simulink model "PC_Quadcopter_Simulation_Hexacopter_health_wind"  (R2022b)
settings: Solver=ode4  StartTime=0.0  StopTime=100  FixedStep=0.01  MaxStep=0.06  RelTol=1e-3
PreLoadFcn:
  | DoB_parameter
model workspace (MAT data in the model file):
  Sig : Simulink.Signal (value not decoded)
values from neighbouring files (symbols this model uses):
  A = [ ... (first row only)    [DoB_parameter.m]
  B = [0 1 0]'    [DoB_parameter.m]
  C = [1 0 0]    [DoB_parameter.m]
  den_Inv_X = conv(num_X,den_Qfilter)    [DoB_parameter.m]
  den_Inv_Y = conv(num_Y, den_Qfilter)    [DoB_parameter.m]
  den_Inv_Z = conv(num_Z, den_Qfilter_Z)    [DoB_parameter.m]
  den_Qfilter = [1 a1/tau a0/tau^2]    [DoB_parameter.m]
  den_Qfilter_Z = [1 a1/tau a0/tau^2]    [DoB_parameter.m]
  I_xx = J(1,1)    [DoB_parameter.m]
  I_yy = J(2,2)    [DoB_parameter.m]
  I_zz = J(3,3)    [DoB_parameter.m]
  IC = block.DialogPrm(2).Data    [quadcopterDynamicsSFunction.m]
  L = [l1 l2 l3]'    [DoB_parameter.m]
  num_Inv_X = conv(den_X,num_Qfilter)    [DoB_parameter.m]
  num_Inv_Y = conv(den_Y, num_Qfilter)    [DoB_parameter.m]
  num_Inv_Z = conv(den_Z, num_Qfilter_Z)    [DoB_parameter.m]
  num_Qfilter = a0/tau^2    (= 100)    [DoB_parameter.m]
  num_Qfilter_Z = a0/tau^2    (= 11.1111111111)    [DoB_parameter.m]
undefined symbols (not defined in the file or in its folder): F, Light, magnitude, MIL, quadModel
libraries: simulink x37, sharedTrackingLibrary x1, aerolibwind2 x1
(part 3 of 3)

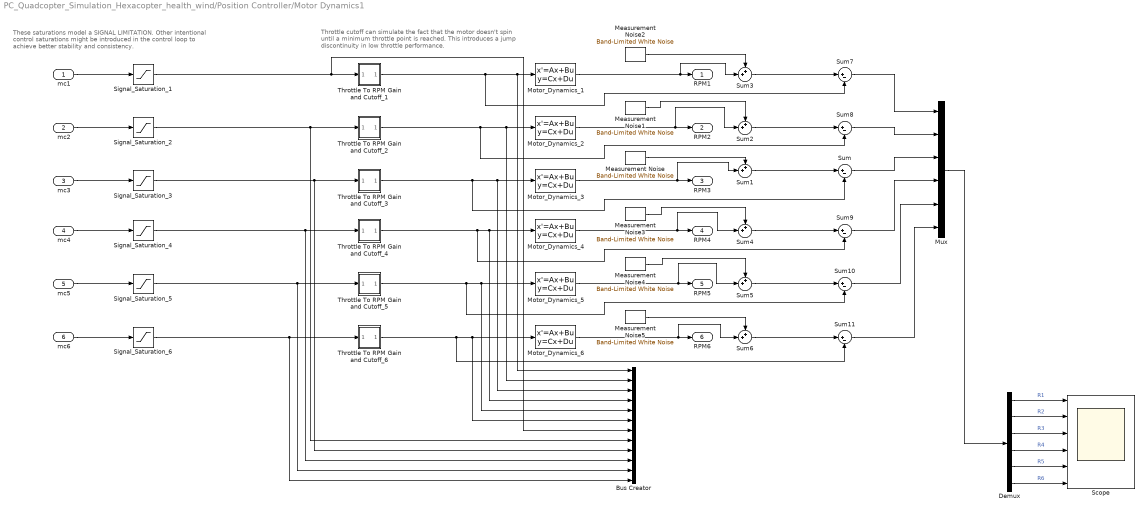
== system PC_Quadcopter_Simulation_Hexacopter_health_wind/Position Controller/Motor Dynamics1 ==
  note: These saturations model a SIGNAL LIMITATION.
      | Other intentional control saturations might be introduced in the
      | control loop to achieve better stability and consistency.
  note: Throttle cutoff can simulate the fact that the motor doesn't
      | spin until a minimum throttle point is reached. This introduces
      | a jump discontinuity in low throttle performance.
  mc1 : Inport
  mc2 : Inport  Port=2
  mc3 : Inport  Port=3
  mc4 : Inport  Port=4
  mc5 : Inport  Port=5
  mc6 : Inport  Port=6
  Bus Creator : BusCreator  Inputs=12
  Demux : Demux  Outputs=6
  Measurement Noise{,1..5} (6 alike) : simulink/Sources/Band-Limited White Noise  Cov=10^2  Ts=0.02  seed=[23342]
  Motor_Dynamics_1 : StateSpace  A=-1/quadModel.T  C=1/quadModel.T  D=0  InitialCondition=IC.w1*quadModel.T
  Motor_Dynamics_2 : StateSpace  A=-1/quadModel.T  C=1/quadModel.T  D=0  InitialCondition=IC.w2*quadModel.T
  Motor_Dynamics_3 : StateSpace  A=-1/quadModel.T  C=1/quadModel.T  D=0  InitialCondition=IC.w3*quadModel.T
  Motor_Dynamics_4 : StateSpace  A=-1/quadModel.T  C=1/quadModel.T  D=0  InitialCondition=IC.w4*quadModel.T
  Motor_Dynamics_5 : StateSpace  A=-1/quadModel.T  C=1/quadModel.T  D=0  InitialCondition=IC.w4*quadModel.T
  Motor_Dynamics_6 : StateSpace  A=-1/quadModel.T  C=1/quadModel.T  D=0  InitialCondition=IC.w4*quadModel.T
  Mux : Mux  Inputs=6
  Scope : Scope  NumInputPorts=6
  Signal_Saturation_{1..6} (6 alike) : Saturate  UpperLimit=100  LowerLimit=0
  Sum{,7..11} (6 alike) : Sum  Inputs=|+-
  Sum{1..6} (6 alike) : Sum  Inputs=++|
  Throttle To RPM Gain and Cutoff_1 : Subsystem
  Throttle To RPM Gain and Cutoff_2 : Subsystem
  Throttle To RPM Gain and Cutoff_3 : Subsystem
  Throttle To RPM Gain and Cutoff_4 : Subsystem
  Throttle To RPM Gain and Cutoff_5 : Subsystem
  Throttle To RPM Gain and Cutoff_6 : Subsystem
  RPM1 : Outport
  RPM2 : Outport  Port=2
  RPM3 : Outport  Port=3
  RPM4 : Outport  Port=4
  RPM5 : Outport  Port=5
  RPM6 : Outport  Port=6
  wires:
  Demux/1 -> Scope/1  "R1"
  Demux/2 -> Scope/2  "R2"
  Demux/3 -> Scope/3  "R3"
  Demux/4 -> Scope/4  "R4"
  Demux/5 -> Scope/5  "R5"
  Demux/6 -> Scope/6  "R6"
  Sum11/1 -> Mux/6
  Sum10/1 -> Mux/5
  Sum9/1 -> Mux/4
  Sum/1 -> Mux/3
  Sum8/1 -> Mux/2
  Sum7/1 -> Mux/1
  Sum6/1 -> Sum11/1
  Sum5/1 -> Sum10/1
  Sum4/1 -> Sum9/1
  Sum3/1 -> Sum7/1
  Sum2/1 -> Sum8/1
  Measurement Noise2/1 -> Sum3/1
  Measurement Noise1/1 -> Sum2/1
  Measurement Noise3/1 -> Sum4/1
  Measurement Noise4/1 -> Sum5/1
  Measurement Noise5/1 -> Sum6/1
  Sum1/1 -> Sum/1
  Measurement Noise/1 -> Sum1/1
  Mux/1 -> Demux/1
  Throttle To RPM Gain and Cutoff_6/1(Out5) -> Bus Creator/6, Motor_Dynamics_6/1, Sum11/2
  Signal_Saturation_6/1 -> Throttle To RPM Gain and Cutoff_6/1(In5), Bus Creator/12
  mc6/1 -> Signal_Saturation_6/1
  Motor_Dynamics_6/1 -> RPM6/1, Sum6/2
  Throttle To RPM Gain and Cutoff_5/1(Out5) -> Bus Creator/5, Motor_Dynamics_5/1, Sum10/2
  Signal_Saturation_5/1 -> Throttle To RPM Gain and Cutoff_5/1(In5), Bus Creator/11
  mc5/1 -> Signal_Saturation_5/1
  Motor_Dynamics_5/1 -> RPM5/1, Sum5/2
  Motor_Dynamics_4/1 -> RPM4/1, Sum4/2
  Motor_Dynamics_3/1 -> RPM3/1, Sum1/2
  Motor_Dynamics_2/1 -> RPM2/1, Sum2/2
  Motor_Dynamics_1/1 -> RPM1/1, Sum3/2
  Throttle To RPM Gain and Cutoff_4/1(Out5) -> Bus Creator/4, Motor_Dynamics_4/1, Sum9/2
  Throttle To RPM Gain and Cutoff_3/1(Out5) -> Bus Creator/3, Motor_Dynamics_3/1, Sum/2
  Throttle To RPM Gain and Cutoff_2/1(Out5) -> Bus Creator/2, Motor_Dynamics_2/1, Sum8/2
  Throttle To RPM Gain and Cutoff_1/1(Out5) -> Motor_Dynamics_1/1, Bus Creator/1, Sum7/2
  Signal_Saturation_4/1 -> Throttle To RPM Gain and Cutoff_4/1(In5), Bus Creator/10
  Signal_Saturation_3/1 -> Throttle To RPM Gain and Cutoff_3/1(In5), Bus Creator/9
  Signal_Saturation_2/1 -> Bus Creator/8, Throttle To RPM Gain and Cutoff_2/1(In5)
  Signal_Saturation_1/1 -> Throttle To RPM Gain and Cutoff_1/1(In5), Bus Creator/7
  mc3/1 -> Signal_Saturation_3/1
  mc2/1 -> Signal_Saturation_2/1
  mc4/1 -> Signal_Saturation_4/1
  mc1/1 -> Signal_Saturation_1/1

== system PC_Quadcopter_Simulation_Hexacopter_health_wind/Position Controller/Phi Command Control ==
  note: -1 Gain is required because a "negative"
      | angle of Phi induces a positive velocity
      | in the body frame y direction!
  Desired Yb Velocity : Inport
  Yb Velocity : Inport  Port=2
  Attitude Limits_Phi : Saturate  UpperLimit=ASat  LowerLimit=-ASat
  Gain : Gain  Gain=-1
  Kdp : Gain  Gain=Kd
  Kpp : Gain  Gain=Kp
  Sum3 : Sum  Inputs=|+-
  Sum6 : Sum  Inputs=|+-
  V Derivative : Derivative
  Phi_cmd : Outport
  wires:
  V Derivative/1 -> Kdp/1
  Attitude Limits_Phi/1 -> Phi_cmd/1  "Phi_cmd"
  Sum6/1 -> Gain/1
  Kpp/1 -> Sum6/1
  Sum3/1 -> Kpp/1  "Velocity Error"
  Yb Velocity/1 -> V Derivative/1, Sum3/2
  Desired Yb Velocity/1 -> Sum3/1
  Gain/1 -> Attitude Limits_Phi/1
  Kdp/1 -> Sum6/2

== system PC_Quadcopter_Simulation_Hexacopter_health_wind/Position Controller/Phi Command Control1 ==
  note: -1 Gain is required because a "negative"
      | angle of Phi induces a positive velocity
      | in the body frame y direction!
  Desired Yb Velocity : Inport
  Attitude Limits_Phi : Saturate  UpperLimit=ASat  LowerLimit=-ASat
  Gain : Gain  Gain=-1
  Kpp : Gain  Gain=Kp
  Phi_cmd : Outport
  wires:
  Gain/1 -> Attitude Limits_Phi/1
  Desired Yb Velocity/1 -> Kpp/1  "Velocity Error"
  Kpp/1 -> Gain/1
  Attitude Limits_Phi/1 -> Phi_cmd/1  "Phi_cmd"

== system PC_Quadcopter_Simulation_Hexacopter_health_wind/Position Controller/Phi Command Control2 ==
  note: -1 Gain is required because a "negative"
      | angle of Phi induces a positive velocity
      | in the body frame y direction!
  Desired Yb Velocity : Inport
  Yb Velocity : Inport  Port=2
  Attitude Limits_Phi : Saturate  UpperLimit=ASat  LowerLimit=-ASat
  Gain : Gain  Gain=-1
  Kdp : Gain  Gain=Kd
  Kpp : Gain  Gain=Kp
  Sum3 : Sum  Inputs=|+-
  Sum6 : Sum  Inputs=|+-
  V Derivative : Derivative
  Phi_cmd : Outport
  wires:
  Kdp/1 -> Sum6/2
  Gain/1 -> Attitude Limits_Phi/1
  Desired Yb Velocity/1 -> Sum3/1
  Yb Velocity/1 -> Sum3/2, V Derivative/1
  Sum3/1 -> Kpp/1  "Velocity Error"
  Kpp/1 -> Sum6/1
  Sum6/1 -> Gain/1
  Attitude Limits_Phi/1 -> Phi_cmd/1  "Phi_cmd"
  V Derivative/1 -> Kdp/1

== system PC_Quadcopter_Simulation_Hexacopter_health_wind/Position Controller/Pitch (Theta) Control ==
  Attitude Command : Inport
  Bus Selector : BusSelector  OutputSignals=The_cmd
  Integrator Limited : Integrator  LimitOutput=on  UpperSaturationLimit=USat  LowerSaturationLimit=LSat
  Kit : Gain  Gain=Kit
  Kpt : Gain  Gain=Kpt
  Sum1 : Sum  Inputs=++|
  Theta Correction : Outport
  wires:
  Attitude Command/1 -> Bus Selector/1
  Sum1/1 -> Theta Correction/1
  Kpt/1 -> Sum1/1  "P Corr"
  Kit/1 -> Sum1/2  "I Corr"
  Integrator Limited/1 -> Kit/1
  Bus Selector/1 -> Integrator Limited/1, Kpt/1  "<The_cmd>"

== system PC_Quadcopter_Simulation_Hexacopter_health_wind/Position Controller/Pitch (Theta) Control1 ==
  Attitude Command : Inport
  Bus Selector : BusSelector  OutputSignals=The_cmd
  Integrator Limited : Integrator  LimitOutput=on  UpperSaturationLimit=USat  LowerSaturationLimit=LSat
  Kit : Gain  Gain=Kit
  Kpt : Gain  Gain=Kpt
  Sum1 : Sum  Inputs=++|
  Theta Correction : Outport
  wires:
  Bus Selector/1 -> Kpt/1, Integrator Limited/1  "<The_cmd>"
  Integrator Limited/1 -> Kit/1
  Kit/1 -> Sum1/2  "I Corr"
  Kpt/1 -> Sum1/1  "P Corr"
  Sum1/1 -> Theta Correction/1
  Attitude Command/1 -> Bus Selector/1

== system PC_Quadcopter_Simulation_Hexacopter_health_wind/Position Controller/Roll (Phi) Control  ==
  "Attitude Command " : Inport
  Bus Selector : BusSelector  OutputSignals=Phi_cmd
  Integrator Limited : Integrator  LimitOutput=on  UpperSaturationLimit=USat  LowerSaturationLimit=LSat
  Kip : Gain  Gain=Kip
  Kpp : Gain  Gain=Kpp
  Sum1 : Sum  Inputs=++|
  Phi Correction : Outport
  wires:
  Sum1/1 -> Phi Correction/1
  Kpp/1 -> Sum1/1  "P Corr"
  Kip/1 -> Sum1/2  "I Corr"
  Integrator Limited/1 -> Kip/1
  "Attitude Command "/1 -> Bus Selector/1
  Bus Selector/1 -> Integrator Limited/1, Kpp/1  "<Phi_cmd>"

== system PC_Quadcopter_Simulation_Hexacopter_health_wind/Position Controller/Roll (Phi) Control 1 ==
  "Attitude Command " : Inport
  Bus Selector : BusSelector  OutputSignals=Phi_cmd
  Integrator Limited : Integrator  LimitOutput=on  UpperSaturationLimit=USat  LowerSaturationLimit=LSat
  Kip : Gain  Gain=Kip
  Kpp : Gain  Gain=Kpp
  Sum1 : Sum  Inputs=++|
  Phi Correction : Outport
  wires:
  Bus Selector/1 -> Kpp/1, Integrator Limited/1  "<Phi_cmd>"
  "Attitude Command "/1 -> Bus Selector/1
  Integrator Limited/1 -> Kip/1
  Kip/1 -> Sum1/2  "I Corr"
  Kpp/1 -> Sum1/1  "P Corr"
  Sum1/1 -> Phi Correction/1

== system PC_Quadcopter_Simulation_Hexacopter_health_wind/Position Controller/Theta Command Control ==
  Desired Xb Velocity : Inport
  Xb Velocity : Inport  Port=2
  Attitude Limits_Theta : Saturate  UpperLimit=ASat  LowerLimit=-ASat
  Kdt : Gain  Gain=Kd
  Kpt : Gain  Gain=Kp
  Sum3 : Sum  Inputs=|+-
  Sum6 : Sum  Inputs=|+-
  U Derivative : Derivative
  The_cmd : Outport
  wires:
  Kdt/1 -> Sum6/2
  U Derivative/1 -> Kdt/1
  Attitude Limits_Theta/1 -> The_cmd/1  "The_cmd"
  Sum6/1 -> Attitude Limits_Theta/1
  Kpt/1 -> Sum6/1
  Sum3/1 -> Kpt/1  "Velocity Error"
  Xb Velocity/1 -> U Derivative/1, Sum3/2
  Desired Xb Velocity/1 -> Sum3/1

== system PC_Quadcopter_Simulation_Hexacopter_health_wind/Position Controller/Theta Command Control1 ==
  Desired Xb Velocity : Inport
  Attitude Limits_Theta : Saturate  UpperLimit=ASat  LowerLimit=-ASat
  Kpt : Gain  Gain=Kp
  The_cmd : Outport
  wires:
  Desired Xb Velocity/1 -> Kpt/1  "Velocity Error"
  Kpt/1 -> Attitude Limits_Theta/1
  Attitude Limits_Theta/1 -> The_cmd/1  "The_cmd"

== system PC_Quadcopter_Simulation_Hexacopter_health_wind/Position Controller/Theta Command Control2 ==
  Desired Xb Velocity : Inport
  Xb Velocity : Inport  Port=2
  Attitude Limits_Theta : Saturate  UpperLimit=ASat  LowerLimit=-ASat
  Kdt : Gain  Gain=Kd
  Kpt : Gain  Gain=Kp
  Sum3 : Sum  Inputs=|+-
  Sum6 : Sum  Inputs=|+-
  U Derivative : Derivative
  The_cmd : Outport
  wires:
  Desired Xb Velocity/1 -> Sum3/1
  Xb Velocity/1 -> Sum3/2, U Derivative/1
  Sum3/1 -> Kpt/1  "Velocity Error"
  Kpt/1 -> Sum6/1
  Sum6/1 -> Attitude Limits_Theta/1
  Attitude Limits_Theta/1 -> The_cmd/1  "The_cmd"
  U Derivative/1 -> Kdt/1
  Kdt/1 -> Sum6/2

== system PC_Quadcopter_Simulation_Hexacopter_health_wind/Position Controller/Yaw (Psi) Control ==
  Attitude Command : Inport
  Bus Selector : BusSelector  OutputSignals=Psi_cmd
  Integrator Limited : Integrator  LimitOutput=on  UpperSaturationLimit=USat  LowerSaturationLimit=LSat
  Kit : Gain  Gain=Kis
  Kps : Gain  Gain=Kps
  Sum1 : Sum  Inputs=++|
  Psi Correction : Outport
  wires:
  Attitude Command/1 -> Bus Selector/1
  Sum1/1 -> Psi Correction/1
  Kps/1 -> Sum1/1  "P Corr"
  Kit/1 -> Sum1/2  "I Corr"
  Integrator Limited/1 -> Kit/1
  Bus Selector/1 -> Integrator Limited/1, Kps/1  "<Psi_cmd>"

== system PC_Quadcopter_Simulation_Hexacopter_health_wind/Position Controller/Yaw (Psi) Control1 ==
  Attitude Command : Inport
  Bus Selector : BusSelector  OutputSignals=Psi_cmd
  Integrator Limited : Integrator  LimitOutput=on  UpperSaturationLimit=USat  LowerSaturationLimit=LSat
  Kit : Gain  Gain=Kis
  Kps : Gain  Gain=Kps
  Sum1 : Sum  Inputs=++|
  Psi Correction : Outport
  wires:
  Bus Selector/1 -> Kps/1, Integrator Limited/1  "<Psi_cmd>"
  Integrator Limited/1 -> Kit/1
  Kit/1 -> Sum1/2  "I Corr"
  Kps/1 -> Sum1/1  "P Corr"
  Sum1/1 -> Psi Correction/1
  Attitude Command/1 -> Bus Selector/1

== system PC_Quadcopter_Simulation_Hexacopter_health_wind/Hexacopter Dynamics/Motor Dynamics/Throttle To RPM Gain and Cutoff_1 ==
  note: minThr should be a quad.mat value
  note: This gain should be a quad.mat value
  note: This constant should be a quad.mat value
  note: Output equals linearly scaled RPM
      | for given throttle input if throttle input >=Throttle Cuttoff (minThr)
      | else output is zero.
  In5 : Inport
  Constant : Constant  Value=quadModel.b
  Gain : Gain  Gain=quadModel.cr
  Minimum Throttle Cutoff : simulink/Logic and Bit Operations/Compare To Constant  relop=>=  const=quadModel.minThr  OutDataTypeStr=uint8
  Product : Product
  Sum1 : Sum  Inputs=++|
  Out5 : Outport
  wires:
  Minimum Throttle Cutoff/1 -> Product/2
  Product/1 -> Out5/1
  In5/1 -> Gain/1, Minimum Throttle Cutoff/1
  Gain/1 -> Sum1/2
  Sum1/1 -> Product/1
  Constant/1 -> Sum1/1

== system PC_Quadcopter_Simulation_Hexacopter_health_wind/Hexacopter Dynamics/Motor Dynamics/Throttle To RPM Gain and Cutoff_2 ==
  note: minThr should be a quad.mat value
  note: This gain should be a quad.mat value
  note: This constant should be a quad.mat value
  note: Output equals linearly scaled RPM
      | for given throttle input if throttle input >=Throttle Cuttoff (minThr)
      | else output is zero.
  In5 : Inport
  Constant : Constant  Value=quadModel.b
  Gain : Gain  Gain=quadModel.cr
  Minimum Throttle Cutoff : simulink/Logic and Bit Operations/Compare To Constant  relop=>=  const=quadModel.minThr  OutDataTypeStr=uint8
  Product : Product
  Sum1 : Sum  Inputs=++|
  Out5 : Outport
  wires:
  Minimum Throttle Cutoff/1 -> Product/2
  Product/1 -> Out5/1
  In5/1 -> Gain/1, Minimum Throttle Cutoff/1
  Gain/1 -> Sum1/2
  Sum1/1 -> Product/1
  Constant/1 -> Sum1/1

== system PC_Quadcopter_Simulation_Hexacopter_health_wind/Hexacopter Dynamics/Motor Dynamics/Throttle To RPM Gain and Cutoff_3 ==
  note: minThr should be a quad.mat value
  note: This gain should be a quad.mat value
  note: This constant should be a quad.mat value
  note: Output equals linearly scaled RPM
      | for given throttle input if throttle input >=Throttle Cuttoff (minThr)
      | else output is zero.
  In5 : Inport
  Constant : Constant  Value=quadModel.b
  Gain : Gain  Gain=quadModel.cr
  Minimum Throttle Cutoff : simulink/Logic and Bit Operations/Compare To Constant  relop=>=  const=quadModel.minThr  OutDataTypeStr=uint8
  Product : Product
  Sum1 : Sum  Inputs=++|
  Out5 : Outport
  wires:
  Minimum Throttle Cutoff/1 -> Product/2
  Product/1 -> Out5/1
  In5/1 -> Gain/1, Minimum Throttle Cutoff/1
  Gain/1 -> Sum1/2
  Sum1/1 -> Product/1
  Constant/1 -> Sum1/1

== system PC_Quadcopter_Simulation_Hexacopter_health_wind/Hexacopter Dynamics/Motor Dynamics/Throttle To RPM Gain and Cutoff_4 ==
  note: minThr should be a quad.mat value
  note: This gain should be a quad.mat value
  note: This constant should be a quad.mat value
  note: Output equals linearly scaled RPM
      | for given throttle input if throttle input >=Throttle Cuttoff (minThr)
      | else output is zero.
  In5 : Inport
  Constant : Constant  Value=quadModel.b
  Gain : Gain  Gain=quadModel.cr
  Minimum Throttle Cutoff : simulink/Logic and Bit Operations/Compare To Constant  relop=>=  const=quadModel.minThr  OutDataTypeStr=uint8
  Product : Product
  Sum1 : Sum  Inputs=++|
  Out5 : Outport
  wires:
  Minimum Throttle Cutoff/1 -> Product/2
  Product/1 -> Out5/1
  In5/1 -> Gain/1, Minimum Throttle Cutoff/1
  Gain/1 -> Sum1/2
  Sum1/1 -> Product/1
  Constant/1 -> Sum1/1

== system PC_Quadcopter_Simulation_Hexacopter_health_wind/Hexacopter Dynamics/Motor Dynamics/Throttle To RPM Gain and Cutoff_5 ==
  note: minThr should be a quad.mat value
  note: This gain should be a quad.mat value
  note: This constant should be a quad.mat value
  note: Output equals linearly scaled RPM
      | for given throttle input if throttle input >=Throttle Cuttoff (minThr)
      | else output is zero.
  In5 : Inport
  Constant : Constant  Value=quadModel.b
  Gain : Gain  Gain=quadModel.cr
  Minimum Throttle Cutoff : simulink/Logic and Bit Operations/Compare To Constant  relop=>=  const=quadModel.minThr  OutDataTypeStr=uint8
  Product : Product
  Sum1 : Sum  Inputs=++|
  Out5 : Outport
  wires:
  Minimum Throttle Cutoff/1 -> Product/2
  Product/1 -> Out5/1
  In5/1 -> Gain/1, Minimum Throttle Cutoff/1
  Gain/1 -> Sum1/2
  Sum1/1 -> Product/1
  Constant/1 -> Sum1/1

== system PC_Quadcopter_Simulation_Hexacopter_health_wind/Hexacopter Dynamics/Motor Dynamics/Throttle To RPM Gain and Cutoff_6 ==
  note: minThr should be a quad.mat value
  note: This gain should be a quad.mat value
  note: This constant should be a quad.mat value
  note: Output equals linearly scaled RPM
      | for given throttle input if throttle input >=Throttle Cuttoff (minThr)
      | else output is zero.
  In5 : Inport
  Constant : Constant  Value=quadModel.b
  Gain : Gain  Gain=quadModel.cr
  Minimum Throttle Cutoff : simulink/Logic and Bit Operations/Compare To Constant  relop=>=  const=quadModel.minThr  OutDataTypeStr=uint8
  Product : Product
  Sum1 : Sum  Inputs=++|
  Out5 : Outport
  wires:
  Minimum Throttle Cutoff/1 -> Product/2
  Product/1 -> Out5/1
  In5/1 -> Gain/1, Minimum Throttle Cutoff/1
  Gain/1 -> Sum1/2
  Sum1/1 -> Product/1
  Constant/1 -> Sum1/1

== system PC_Quadcopter_Simulation_Hexacopter_health_wind/Hexacopter Dynamics/a_x, a_y, a_z/Subsystem ==
  q : Inport
  r : Inport  Port=2
  U : Inport  Port=3
  V : Inport  Port=4
  W : Inport  Port=5
  Theta : Inport  Port=6
  Constant : Constant  Value=quadModel.g
  Cos : Trigonometry
  Derivative : Derivative
  Product : Product
  Product1 : Product
  Product2 : Product
  Sum : Sum  Inputs=+--
  Sum1 : Sum  Inputs=|++
  a_x : Outport
  wires:
  Theta/1 -> Cos/1
  Cos/1 -> Product/1
  Constant/1 -> Product/2
  Product1/1 -> Sum1/1
  Derivative/1 -> Sum1/2
  Sum1/1 -> Sum/1
  Sum/1 -> a_x/1
  Product2/1 -> Sum/2
  Product/1 -> Sum/3
  U/1 -> Derivative/1
  q/1 -> Product1/1
  W/1 -> Product1/2
  r/1 -> Product2/1
  V/1 -> Product2/2

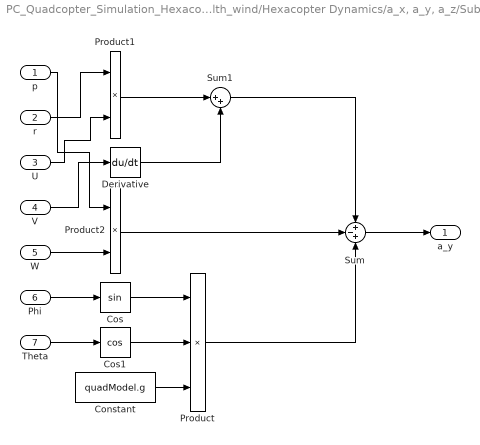
== system PC_Quadcopter_Simulation_Hexacopter_health_wind/Hexacopter Dynamics/a_x, a_y, a_z/Subsystem1 ==
  p : Inport
  r : Inport  Port=2
  U : Inport  Port=3
  V : Inport  Port=4
  W : Inport  Port=5
  Phi : Inport  Port=6
  Theta : Inport  Port=7
  Constant : Constant  Value=quadModel.g
  Cos : Trigonometry
  Cos1 : Trigonometry  Operator=cos
  Derivative : Derivative
  Product : Product  Inputs=3
  Product1 : Product
  Product2 : Product
  Sum : Sum  Inputs=+-+
  Sum1 : Sum  Inputs=|++
  a_y : Outport
  wires:
  V/1 -> Derivative/1
  Theta/1 -> Cos1/1
  Phi/1 -> Cos/1
  Cos/1 -> Product/1
  Cos1/1 -> Product/2
  Constant/1 -> Product/3
  Derivative/1 -> Sum1/2
  r/1 -> Product1/1
  U/1 -> Product1/2
  W/1 -> Product2/2
  p/1 -> Product2/1
  Product1/1 -> Sum1/1
  Product2/1 -> Sum/2
  Sum1/1 -> Sum/1
  Product/1 -> Sum/3
  Sum/1 -> a_y/1

== system PC_Quadcopter_Simulation_Hexacopter_health_wind/Hexacopter Dynamics/a_x, a_y, a_z/Subsystem2 ==
  p : Inport
  q : Inport  Port=2
  U : Inport  Port=3
  V : Inport  Port=4
  W : Inport  Port=5
  Phi : Inport  Port=6
  Theta : Inport  Port=7
  Constant1 : Constant  Value=quadModel.g
  Cos : Trigonometry  Operator=cos
  Cos1 : Trigonometry  Operator=cos
  Derivative : Derivative
  Product : Product  Inputs=3
  Product1 : Product
  Product2 : Product
  Sum : Sum  Inputs=+-+
  Sum1 : Sum  Inputs=|++
  a_z : Outport
  wires:
  Cos1/1 -> Product/2
  Constant1/1 -> Product/3
  Cos/1 -> Product/1
  Sum/1 -> a_z/1
  Theta/1 -> Cos1/1
  Phi/1 -> Cos/1
  W/1 -> Derivative/1
  p/1 -> Product1/1
  V/1 -> Product1/2
  q/1 -> Product2/1
  U/1 -> Product2/2
  Product1/1 -> Sum1/1
  Derivative/1 -> Sum1/2
  Product2/1 -> Sum/2
  Sum1/1 -> Sum/1
  Product/1 -> Sum/3

== system PC_Quadcopter_Simulation_Hexacopter_health_wind/Position Controller/Motor Dynamics/Throttle To RPM Gain and Cutoff_1 ==
  note: minThr should be a quad.mat value
  note: This gain should be a quad.mat value
  note: This constant should be a quad.mat value
  note: Output equals linearly scaled RPM
      | for given throttle input if throttle input >=Throttle Cuttoff (minThr)
      | else output is zero.
  In5 : Inport
  Constant : Constant  Value=quadModel.b
  Gain : Gain  Gain=quadModel.cr
  Minimum Throttle Cutoff : simulink/Logic and Bit Operations/Compare To Constant  relop=>=  const=quadModel.minThr  OutDataTypeStr=uint8
  Product : Product
  Sum1 : Sum  Inputs=++|
  Out5 : Outport
  wires:
  Minimum Throttle Cutoff/1 -> Product/2
  Product/1 -> Out5/1
  In5/1 -> Gain/1, Minimum Throttle Cutoff/1
  Gain/1 -> Sum1/2
  Sum1/1 -> Product/1
  Constant/1 -> Sum1/1

== system PC_Quadcopter_Simulation_Hexacopter_health_wind/Position Controller/Motor Dynamics/Throttle To RPM Gain and Cutoff_2 ==
  note: minThr should be a quad.mat value
  note: This gain should be a quad.mat value
  note: This constant should be a quad.mat value
  note: Output equals linearly scaled RPM
      | for given throttle input if throttle input >=Throttle Cuttoff (minThr)
      | else output is zero.
  In5 : Inport
  Constant : Constant  Value=quadModel.b
  Gain : Gain  Gain=quadModel.cr
  Minimum Throttle Cutoff : simulink/Logic and Bit Operations/Compare To Constant  relop=>=  const=quadModel.minThr  OutDataTypeStr=uint8
  Product : Product
  Sum1 : Sum  Inputs=++|
  Out5 : Outport
  wires:
  Minimum Throttle Cutoff/1 -> Product/2
  Product/1 -> Out5/1
  In5/1 -> Gain/1, Minimum Throttle Cutoff/1
  Gain/1 -> Sum1/2
  Sum1/1 -> Product/1
  Constant/1 -> Sum1/1

== system PC_Quadcopter_Simulation_Hexacopter_health_wind/Position Controller/Motor Dynamics/Throttle To RPM Gain and Cutoff_3 ==
  note: minThr should be a quad.mat value
  note: This gain should be a quad.mat value
  note: This constant should be a quad.mat value
  note: Output equals linearly scaled RPM
      | for given throttle input if throttle input >=Throttle Cuttoff (minThr)
      | else output is zero.
  In5 : Inport
  Constant : Constant  Value=quadModel.b
  Gain : Gain  Gain=quadModel.cr
  Minimum Throttle Cutoff : simulink/Logic and Bit Operations/Compare To Constant  relop=>=  const=quadModel.minThr  OutDataTypeStr=uint8
  Product : Product
  Sum1 : Sum  Inputs=++|
  Out5 : Outport
  wires:
  Minimum Throttle Cutoff/1 -> Product/2
  Product/1 -> Out5/1
  In5/1 -> Gain/1, Minimum Throttle Cutoff/1
  Gain/1 -> Sum1/2
  Sum1/1 -> Product/1
  Constant/1 -> Sum1/1

== system PC_Quadcopter_Simulation_Hexacopter_health_wind/Position Controller/Motor Dynamics/Throttle To RPM Gain and Cutoff_4 ==
  note: minThr should be a quad.mat value
  note: This gain should be a quad.mat value
  note: This constant should be a quad.mat value
  note: Output equals linearly scaled RPM
      | for given throttle input if throttle input >=Throttle Cuttoff (minThr)
      | else output is zero.
  In5 : Inport
  Constant : Constant  Value=quadModel.b
  Gain : Gain  Gain=quadModel.cr
  Minimum Throttle Cutoff : simulink/Logic and Bit Operations/Compare To Constant  relop=>=  const=quadModel.minThr  OutDataTypeStr=uint8
  Product : Product
  Sum1 : Sum  Inputs=++|
  Out5 : Outport
  wires:
  Minimum Throttle Cutoff/1 -> Product/2
  Product/1 -> Out5/1
  In5/1 -> Gain/1, Minimum Throttle Cutoff/1
  Gain/1 -> Sum1/2
  Sum1/1 -> Product/1
  Constant/1 -> Sum1/1

== system PC_Quadcopter_Simulation_Hexacopter_health_wind/Position Controller/Motor Dynamics/Throttle To RPM Gain and Cutoff_5 ==
  note: minThr should be a quad.mat value
  note: This gain should be a quad.mat value
  note: This constant should be a quad.mat value
  note: Output equals linearly scaled RPM
      | for given throttle input if throttle input >=Throttle Cuttoff (minThr)
      | else output is zero.
  In5 : Inport
  Constant : Constant  Value=quadModel.b
  Gain : Gain  Gain=quadModel.cr
  Minimum Throttle Cutoff : simulink/Logic and Bit Operations/Compare To Constant  relop=>=  const=quadModel.minThr  OutDataTypeStr=uint8
  Product : Product
  Sum1 : Sum  Inputs=++|
  Out5 : Outport
  wires:
  Minimum Throttle Cutoff/1 -> Product/2
  Product/1 -> Out5/1
  In5/1 -> Gain/1, Minimum Throttle Cutoff/1
  Gain/1 -> Sum1/2
  Sum1/1 -> Product/1
  Constant/1 -> Sum1/1

== system PC_Quadcopter_Simulation_Hexacopter_health_wind/Position Controller/Motor Dynamics/Throttle To RPM Gain and Cutoff_6 ==
  note: minThr should be a quad.mat value
  note: This gain should be a quad.mat value
  note: This constant should be a quad.mat value
  note: Output equals linearly scaled RPM
      | for given throttle input if throttle input >=Throttle Cuttoff (minThr)
      | else output is zero.
  In5 : Inport
  Constant : Constant  Value=quadModel.b
  Gain : Gain  Gain=quadModel.cr
  Minimum Throttle Cutoff : simulink/Logic and Bit Operations/Compare To Constant  relop=>=  const=quadModel.minThr  OutDataTypeStr=uint8
  Product : Product
  Sum1 : Sum  Inputs=++|
  Out5 : Outport
  wires:
  Minimum Throttle Cutoff/1 -> Product/2
  Product/1 -> Out5/1
  In5/1 -> Gain/1, Minimum Throttle Cutoff/1
  Gain/1 -> Sum1/2
  Sum1/1 -> Product/1
  Constant/1 -> Sum1/1

== system PC_Quadcopter_Simulation_Hexacopter_health_wind/Position Controller/Motor Dynamics1/Throttle To RPM Gain and Cutoff_1 ==
  note: Output equals linearly scaled RPM
      | for given throttle input if throttle input >=Throttle Cuttoff (minThr)
      | else output is zero.
  note: This constant should be a quad.mat value
  note: This gain should be a quad.mat value
  note: minThr should be a quad.mat value
  In5 : Inport
  Constant : Constant  Value=quadModel.b
  Gain : Gain  Gain=quadModel.cr
  Minimum Throttle Cutoff : simulink/Logic and Bit Operations/Compare To Constant  relop=>=  const=quadModel.minThr  OutDataTypeStr=uint8
  Product : Product
  Sum1 : Sum  Inputs=++|
  Out5 : Outport
  wires:
  Constant/1 -> Sum1/1
  Sum1/1 -> Product/1
  Gain/1 -> Sum1/2
  In5/1 -> Minimum Throttle Cutoff/1, Gain/1
  Product/1 -> Out5/1
  Minimum Throttle Cutoff/1 -> Product/2

== system PC_Quadcopter_Simulation_Hexacopter_health_wind/Position Controller/Motor Dynamics1/Throttle To RPM Gain and Cutoff_2 ==
  note: Output equals linearly scaled RPM
      | for given throttle input if throttle input >=Throttle Cuttoff (minThr)
      | else output is zero.
  note: This constant should be a quad.mat value
  note: This gain should be a quad.mat value
  note: minThr should be a quad.mat value
  In5 : Inport
  Constant : Constant  Value=quadModel.b
  Gain : Gain  Gain=quadModel.cr
  Minimum Throttle Cutoff : simulink/Logic and Bit Operations/Compare To Constant  relop=>=  const=quadModel.minThr  OutDataTypeStr=uint8
  Product : Product
  Sum1 : Sum  Inputs=++|
  Out5 : Outport
  wires:
  Constant/1 -> Sum1/1
  Sum1/1 -> Product/1
  Gain/1 -> Sum1/2
  In5/1 -> Minimum Throttle Cutoff/1, Gain/1
  Product/1 -> Out5/1
  Minimum Throttle Cutoff/1 -> Product/2

== system PC_Quadcopter_Simulation_Hexacopter_health_wind/Position Controller/Motor Dynamics1/Throttle To RPM Gain and Cutoff_3 ==
  note: Output equals linearly scaled RPM
      | for given throttle input if throttle input >=Throttle Cuttoff (minThr)
      | else output is zero.
  note: This constant should be a quad.mat value
  note: This gain should be a quad.mat value
  note: minThr should be a quad.mat value
  In5 : Inport
  Constant : Constant  Value=quadModel.b
  Gain : Gain  Gain=quadModel.cr
  Minimum Throttle Cutoff : simulink/Logic and Bit Operations/Compare To Constant  relop=>=  const=quadModel.minThr  OutDataTypeStr=uint8
  Product : Product
  Sum1 : Sum  Inputs=++|
  Out5 : Outport
  wires:
  Constant/1 -> Sum1/1
  Sum1/1 -> Product/1
  Gain/1 -> Sum1/2
  In5/1 -> Minimum Throttle Cutoff/1, Gain/1
  Product/1 -> Out5/1
  Minimum Throttle Cutoff/1 -> Product/2

== system PC_Quadcopter_Simulation_Hexacopter_health_wind/Position Controller/Motor Dynamics1/Throttle To RPM Gain and Cutoff_4 ==
  note: Output equals linearly scaled RPM
      | for given throttle input if throttle input >=Throttle Cuttoff (minThr)
      | else output is zero.
  note: This constant should be a quad.mat value
  note: This gain should be a quad.mat value
  note: minThr should be a quad.mat value
  In5 : Inport
  Constant : Constant  Value=quadModel.b
  Gain : Gain  Gain=quadModel.cr
  Minimum Throttle Cutoff : simulink/Logic and Bit Operations/Compare To Constant  relop=>=  const=quadModel.minThr  OutDataTypeStr=uint8
  Product : Product
  Sum1 : Sum  Inputs=++|
  Out5 : Outport
  wires:
  Constant/1 -> Sum1/1
  Sum1/1 -> Product/1
  Gain/1 -> Sum1/2
  In5/1 -> Minimum Throttle Cutoff/1, Gain/1
  Product/1 -> Out5/1
  Minimum Throttle Cutoff/1 -> Product/2

== system PC_Quadcopter_Simulation_Hexacopter_health_wind/Position Controller/Motor Dynamics1/Throttle To RPM Gain and Cutoff_5 ==
  note: Output equals linearly scaled RPM
      | for given throttle input if throttle input >=Throttle Cuttoff (minThr)
      | else output is zero.
  note: This constant should be a quad.mat value
  note: This gain should be a quad.mat value
  note: minThr should be a quad.mat value
  In5 : Inport
  Constant : Constant  Value=quadModel.b
  Gain : Gain  Gain=quadModel.cr
  Minimum Throttle Cutoff : simulink/Logic and Bit Operations/Compare To Constant  relop=>=  const=quadModel.minThr  OutDataTypeStr=uint8
  Product : Product
  Sum1 : Sum  Inputs=++|
  Out5 : Outport
  wires:
  Constant/1 -> Sum1/1
  Sum1/1 -> Product/1
  Gain/1 -> Sum1/2
  In5/1 -> Minimum Throttle Cutoff/1, Gain/1
  Product/1 -> Out5/1
  Minimum Throttle Cutoff/1 -> Product/2

== system PC_Quadcopter_Simulation_Hexacopter_health_wind/Position Controller/Motor Dynamics1/Throttle To RPM Gain and Cutoff_6 ==
  note: Output equals linearly scaled RPM
      | for given throttle input if throttle input >=Throttle Cuttoff (minThr)
      | else output is zero.
  note: This constant should be a quad.mat value
  note: This gain should be a quad.mat value
  note: minThr should be a quad.mat value
  In5 : Inport
  Constant : Constant  Value=quadModel.b
  Gain : Gain  Gain=quadModel.cr
  Minimum Throttle Cutoff : simulink/Logic and Bit Operations/Compare To Constant  relop=>=  const=quadModel.minThr  OutDataTypeStr=uint8
  Product : Product
  Sum1 : Sum  Inputs=++|
  Out5 : Outport
  wires:
  Constant/1 -> Sum1/1
  Sum1/1 -> Product/1
  Gain/1 -> Sum1/2
  In5/1 -> Minimum Throttle Cutoff/1, Gain/1
  Product/1 -> Out5/1
  Minimum Throttle Cutoff/1 -> Product/2

== matlab function PC_Quadcopter_Simulation_Hexacopter_health_wind/Position Controller/Hexacopter Control Mixing1/MATLAB Function ==
  data: u input; y output
function y = fcn(u)
%% mixing matrix: PID correction to motors
m = 1.023;
g = 9.81;
ct = 1.4865e-07;
cr = 80.5840;
b = 976.2;
%% health state 6*1
h = u(5:10,1);
FDI = u(11,1);
% 
% A = [
%     -1/h(1,1) -1/h(1,1) -1/h(1,1) 1/h(1,1)
%     1/h(2,1) -1/h(2,1) 1/h(2,1) 1/h(2,1)
%     1/h(3,1) 0 -1/h(3,1) 1/h(3,1)
%     1/h(4,1) 1/h(4,1) 1/h(4,1) 1/h(4,1)
%     -1/h(5,1) 1/h(5,1) -1/h(5,1) 1/h(5,1)
%     -1/h(6,1) 0 1/h(6,1) 1/h(6,1)
%     ];

A = [
    -1 -1 -1 1
    1 -1 1 1
    1 0 -1 1
    1 1 1 1
    -1 1 -1 1
    -1 0 1 1
    ];

%% 고장을 고려한 mixing 변화
if FDI==1 | FDI==4
h(1,1)=0;
h(2,1)=1;
h(3,1)=1;
h(4,1)=0;
h(5,1)=1;
h(6,1)=1;

A = [
    -1 -1 -1 1
    1 -1 1 1
    1 0 -1 1
    1 1 1 1
    -1 1 -1 1
    -1 0 1 1
    ];

elseif FDI==2 | FDI==5
h(1,1)=1;
h(2,1)=0;
h(3,1)=1;
h(4,1)=1;
h(5,1)=0;
h(6,1)=1;

A = [
    -1 -1 -1 1
    1 -1 1 1
    1 0 -1 1
    1 1 1 1
    -1 1 -1 1
    -1 0 1 1
    ];

elseif FDI==3 | FDI==6
h(1,1)=1;
h(2,1)=1;
h(3,1)=0;
h(4,1)=1;
h(5,1)=1;
h(6,1)=0;
% 
A = [
    -1 -1 -1 1
    1 -1 1 1
    1 0 -1 1
    1 1 1 1
    -1 1 -1 1
    -1 0 1 1
    ];

end
for i=1:6
    A(i,:) = h(i)*A(i,:);
end

%% 고장을 고려한 건강한 모터의 추력 증가
% A = sqrt(6/sum(h))*A;


y = A*( u(1:4,:) )
% y = A*( u(1:4,:) ) + (sqrt(m*g/sum(h)/ct)-b)/cr ...
%     - (sqrt(m*g/6/ct)-b)/cr ;

== matlab function PC_Quadcopter_Simulation_Hexacopter_health_wind/Fault Diagnosis/Generate Residual/MATLAB Function - Generate Predicted Output ==
  data: xEstimated input; yPredicted output; u input
function yPredicted = generatePredictedOutput(xEstimated,u)

%   Copyright 2017 The MathWorks, Inc.

%#codegen

% Given state estimates at previous time (k-1) utilizing measurements up to
% (k-1), predict states at current step.
xPredicted = myStateTransitionFcn(xEstimated,u); % xhat[k|k-1]
% Generate output estimate, again without utilizing the measurement at
% current time.
yPredicted = myMeasurementFcn(xPredicted); % y[k|k-1]
end

== matlab function PC_Quadcopter_Simulation_Hexacopter_health_wind/Hexacopter Control Mixing/MATLAB Function ==
  data: u input; y output
function y = fcn(u)
%% mixing matrix: PID correction to motors
m = 1.023;
g = 9.81;
ct = 1.4865e-07;
cr = 80.5840;
b = 976.2;
%% health state 6*1
h = u(5:10,1);
FDI = u(11,1);
% 
% A = [
%     -1/h(1,1) -1/h(1,1) -1/h(1,1) 1/h(1,1)
%     1/h(2,1) -1/h(2,1) 1/h(2,1) 1/h(2,1)
%     1/h(3,1) 0 -1/h(3,1) 1/h(3,1)
%     1/h(4,1) 1/h(4,1) 1/h(4,1) 1/h(4,1)
%     -1/h(5,1) 1/h(5,1) -1/h(5,1) 1/h(5,1)
%     -1/h(6,1) 0 1/h(6,1) 1/h(6,1)
%     ];

A = [
    -1 -1 -1 1
    1 -1 1 1
    1 0 -1 1
    1 1 1 1
    -1 1 -1 1
    -1 0 1 1
    ];

%% 고장을 고려한 mixing 변화
if FDI==1 | FDI==4
h(1,1)=0;
h(2,1)=1;
h(3,1)=1;
h(4,1)=0;
h(5,1)=1;
h(6,1)=1;

A = [
    -1 -1 -1 1
    1 -1 1 1
    1 0 -1 1
    1 1 1 1
    -1 1 -1 1
    -1 0 1 1
    ];

elseif FDI==2 | FDI==5
h(1,1)=1;
h(2,1)=0;
h(3,1)=1;
h(4,1)=1;
h(5,1)=0;
h(6,1)=1;

A = [
    -1 -1 -1 1
    1 -1 1 1
    1 0 -1 1
    1 1 1 1
    -1 1 -1 1
    -1 0 1 1
    ];

elseif FDI==3 | FDI==6
h(1,1)=1;
h(2,1)=1;
h(3,1)=0;
h(4,1)=1;
h(5,1)=1;
h(6,1)=0;
% 
A = [
    -1 -1 -1 1
    1 -1 1 1
    1 0 -1 1
    1 1 1 1
    -1 1 -1 1
    -1 0 1 1
    ];

end
for i=1:6
    A(i,:) = h(i)*A(i,:);
end

%% 고장을 고려한 건강한 모터의 추력 증가
% A = sqrt(6/sum(h))*A;


y = A*( u(1:4,:) )
% y = A*( u(1:4,:) ) + (sqrt(m*g/sum(h)/ct)-b)/cr ...
%     - (sqrt(m*g/6/ct)-b)/cr ;

== matlab function PC_Quadcopter_Simulation_Hexacopter_health_wind/Fault Diagnosis/MATLAB Function ==
  data: p input; y output; q input; r input; a_z input; Z input; h input; t input
function y = FDI(p,q,r,a_z,Z,h,t)
% th = 0.04;
p_th = 0.03;
q_th = 0.07;
r_th = 0.015;
% z_th = 0.001;
%  & a_z<-z_th
y=0;

while y==0
    if  Z>0 & p>p_th & q>q_th & r>r_th & h(1) < 0.88 | t>0.2 & h(1) < 0.6
        y=1;
    elseif Z>0 & p<-p_th & q>q_th & r<-r_th & h(2) < 0.88 | t>0.2 & h(2) < 0.6
        y=2;
    elseif Z>0 & p<-p_th & -q_th<q & q<q_th & r>r_th & h(3) < 0.88 | t>0.2 & h(3) < 0.6
        y=3;
    elseif Z>0 & p<-p_th & q<-q_th & r<-r_th & h(4) < 0.88 | t>0.2 & h(4) < 0.6
        y=4;
    elseif Z>0 & p>p_th & q<-q_th & r>r_th & h(5) < 0.88 | t>0.2 & h(5) < 0.6
        y=5;
%     elseif Z>0 & p>p_th & -q_th<q & q<q_th & r<-r_th  & h(6) < 0.88 | t>0.2 & h(6) < 0.6
%         y=6;
    end
    break
end            
end

== matlab function PC_Quadcopter_Simulation_Hexacopter_health_wind/Fault Diagnosis/MATLAB Function1 ==
  data: R1 input; y output; R2 input; R3 input; R4 input; R5 input; R6 input; Z input; h input; t input
function y = FDI(R1,R2,R3,R4,R5,R6,Z,h,t)
% th = 0.04;
RPM_th = 1000;

y=0;

while y==0
    if  Z>0 & t>0.5 & R1>RPM_th & h(1) < 0.6 
%         | t>0.2 & h(1) < 0.55
        y=1;
    elseif Z>0 & t>0.5 & R2>RPM_th & h(2) < 0.6 
        y=2;
    elseif Z>0 & t>0.5 & R3>RPM_th & h(3) < 0.6 
%         | t>0.5 & h(3) < 0.6
        y=3;
    elseif Z>0 & t>0.5 & R4>RPM_th & h(4) < 0.6 
        y=4;
    elseif Z>0 & t>0.5 & R5>RPM_th & h(5) < 0.6 
        y=5;
%     elseif Z>0 & t>0.5 & R6>RPM_th & h(6) < 0.6 | Z>0 & t>0.5 & R6<-RPM_th & h(6) < 0.6
%         y=6;
    end
    break
end            
end

== matlab function PC_Quadcopter_Simulation_Hexacopter_health_wind/Position Controller/Hexacopter Control Mixing/MATLAB Function ==
  data: u input; y output
function y = fcn(u)
%% mixing matrix: PID correction to motors
m = 1.023;
g = 9.81;
ct = 1.4865e-07;
cr = 80.5840;
b = 976.2;
%% health state 6*1
h = u(5:10,1);
FDI = u(11,1);
% 
% A = [
%     -1/h(1,1) -1/h(1,1) -1/h(1,1) 1/h(1,1)
%     1/h(2,1) -1/h(2,1) 1/h(2,1) 1/h(2,1)
%     1/h(3,1) 0 -1/h(3,1) 1/h(3,1)
%     1/h(4,1) 1/h(4,1) 1/h(4,1) 1/h(4,1)
%     -1/h(5,1) 1/h(5,1) -1/h(5,1) 1/h(5,1)
%     -1/h(6,1) 0 1/h(6,1) 1/h(6,1)
%     ];

A = [
    -1 -1 -1 1
    1 -1 1 1
    1 0 -1 1
    1 1 1 1
    -1 1 -1 1
    -1 0 1 1
    ];

%% 고장을 고려한 mixing 변화
if FDI==1 | FDI==4
h(1,1)=0;
h(2,1)=1;
h(3,1)=1;
h(4,1)=0;
h(5,1)=1;
h(6,1)=1;

A = [
    -1 -1 -1 1
    1 -1 1 1
    1 0 -1 1
    1 1 1 1
    -1 1 -1 1
    -1 0 1 1
    ];

elseif FDI==2 | FDI==5
h(1,1)=1;
h(2,1)=0;
h(3,1)=1;
h(4,1)=1;
h(5,1)=0;
h(6,1)=1;

A = [
    -1 -1 -1 1
    1 -1 1 1
    1 0 -1 1
    1 1 1 1
    -1 1 -1 1
    -1 0 1 1
    ];

elseif FDI==3 | FDI==6
h(1,1)=1;
h(2,1)=1;
h(3,1)=0;
h(4,1)=1;
h(5,1)=1;
h(6,1)=0;
% 
A = [
    -1 -1 -1 1
    1 -1 1 1
    1 0 -1 1
    1 1 1 1
    -1 1 -1 1
    -1 0 1 1
    ];

end
for i=1:6
    A(i,:) = h(i)*A(i,:);
end

%% 고장을 고려한 건강한 모터의 추력 증가
% A = sqrt(6/sum(h))*A;


y = A*( u(1:4,:) )
% y = A*( u(1:4,:) ) + (sqrt(m*g/sum(h)/ct)-b)/cr ...
%     - (sqrt(m*g/6/ct)-b)/cr ;

== matlab function PC_Quadcopter_Simulation_Hexacopter_health_wind/Hexacopter Dynamics/MATLAB Function ==
  data: u input; y output
function y = fcn(u)
psi = u;

y = [cos(psi) sin(psi) 0;
     -sin(psi) cos(psi) 0;
        0   0   1];

== matlab function PC_Quadcopter_Simulation_Hexacopter_health_wind/Hexacopter Dynamics/MATLAB Function1 ==
  data: u input; y output
function y = fcn(u)
theta = u;
y = [cos(theta) 0 -sin(theta);
     0 1 0;
     sin(theta) 0 cos(theta)];

== matlab function PC_Quadcopter_Simulation_Hexacopter_health_wind/Hexacopter Dynamics/MATLAB Function2 ==
  data: u input; y output
function y = fcn(u)
phi = u;
y = [1 0 0;
     0  cos(phi) sin(phi);
     0 -sin(phi) cos(phi)];

== matlab function PC_Quadcopter_Simulation_Hexacopter_health_wind/Hexacopter Dynamics/MATLAB Function3 ==
  data: u input; y output; v input; w input
function y = fcn(u,v,w)

y = sqrt(u.^2+v.^2+w.^2);

== matlab function PC_Quadcopter_Simulation_Hexacopter_health_wind/Hexacopter Dynamics/MATLAB Function4 ==
  data: a input; y output; b input; c input
function y = fcn(a,b,c)

y = a*b*c;
